simulink model "soc_rfsoc_fpga"  (R2025b)
settings: Solver=FixedStepDiscrete  StartTime=0.0  StopTime=15e-4  RelTol=1e-3
undefined symbols (not defined in the file): downSamplingFactor, SampleTime
libraries: simulink x4, hdlsllib x3, hwlogicconnlib x2, dspsrcs4 x2, socmemlib x1
settings Model: DataTypeOverride=Off  Creator=The MathWorks, Inc.  LastModifiedBy=The MathWorks, Inc.
settings SolverCC: AlgebraicLoopSolver=TrustRegion  PositivePriorityOrder=on  MaxZcPerStep=1.0
settings DataIOCC: SaveOutput=off  SaveTime=off  ReturnWorkspaceOutputs=off
settings OptimizationCC: BlockReduction=off  ConditionallyExecuteInputs=off  DefaultParameterBehavior=Inlined  PassReuseOutputArgsAs=Individual arguments  MaxStackSize=64  EfficientTunableParamExpr=on
settings DebuggingCC: AlgebraicLoopMsg=error  SingleTaskRateTransMsg=error  IntegerOverflowMsg=none  ParameterPrecisionLossMsg=none  ParameterTunabilityLossMsg=error  UnconnectedInputMsg=warning  UnconnectedOutputMsg=warning  UnconnectedLineMsg=warning  PregeneratedLibrarySubsystemCodeDiagnostic=none  SFUnexpectedBacktrackingDiag=warning  SFNoUnconditionalDefaultTransitionDiag=warning  ArithmeticOperatorsInVariantConditions=warning
settings HardwareCC: ProdBitPerPointer=32.0  ProdBitPerSizeT=32.0  ProdBitPerPtrDiffT=32.0  ProdLargestAtomicFloat=None  ProdIntDivRoundTo=Undefined  ProdEndianess=Unspecified  ProdWordSize=32.0  ProdHWDeviceType=ASIC/FPGA->ASIC/FPGA  TargetBitPerLong=64.0  TargetBitPerPointer=64.0  TargetBitPerSizeT=64.0  TargetBitPerPtrDiffT=64.0  TargetLongLongMode=on  TargetIntDivRoundTo=Zero  TargetEndianess=LittleEndian  TargetWordSize=64.0  TargetHWDeviceType=Custom Processor->MATLAB Host Computer  ProdEqTarget=off  HardwareBoardFeatureSet=SoCBlockset
settings ModelReferenceCC: EnableRefExpFcnMdlSchedulingChecks=on  ModelReferenceNumInstancesAllowed=Single
settings SFSimCC: SimUseLocalCustomCode=off
settings RTWCC: SystemTargetFile=ert.tlc  HardwareBoard=Xilinx Zynq UltraScale+ RFSoC ZCU111 Evaluation Kit  TLCOptions="-aInlineSetEventsForThisBaseRateFcn=TLC_FALSE -aSuppressMultiTaskScheduler=TLC_FALSE  -aRateBasedStepFcn=0"  TemplateMakefile=ert_default_tmf  GenerateReport=on  RTWUseLocalCustomCode=off  Toolchain=Linaro AArch64 Linux v6.3.1  IncludeHyperlinkInReport=on  LaunchReport=on  GenerateTraceInfo=on  GenerateTraceReport=on  GenerateTraceReportSl=on  GenerateTraceReportSf=on  GenerateTraceReportEml=on  GPUComputeCapability=3.5  DLArmComputeVersion=19.05  Description=Embedded Coder
settings CodeAppCC: ForceParamTrailComments=on  IgnoreCustomStorageClasses=off  OperatorAnnotations=on  SimulinkDataObjDesc=on  SFDataObjDesc=on  InsertBlockDesc=on
settings ERTTargetCC: InlinedParameterPlacement=Hierarchical  DynamicArrayContainerType=coder::array  SubcomponentCodeInterfacePackaging=Nonreusable function

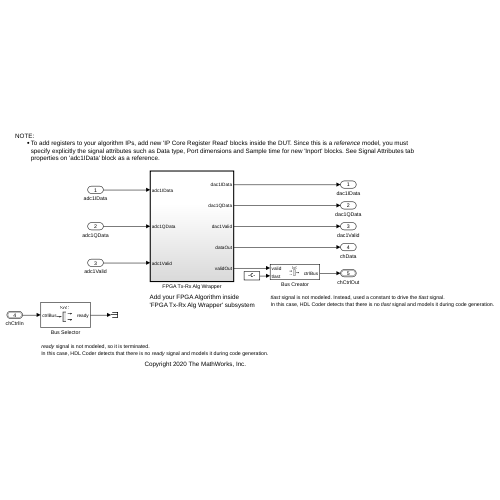
[thumbnail: Simulink's stored preview of the top-level diagram]
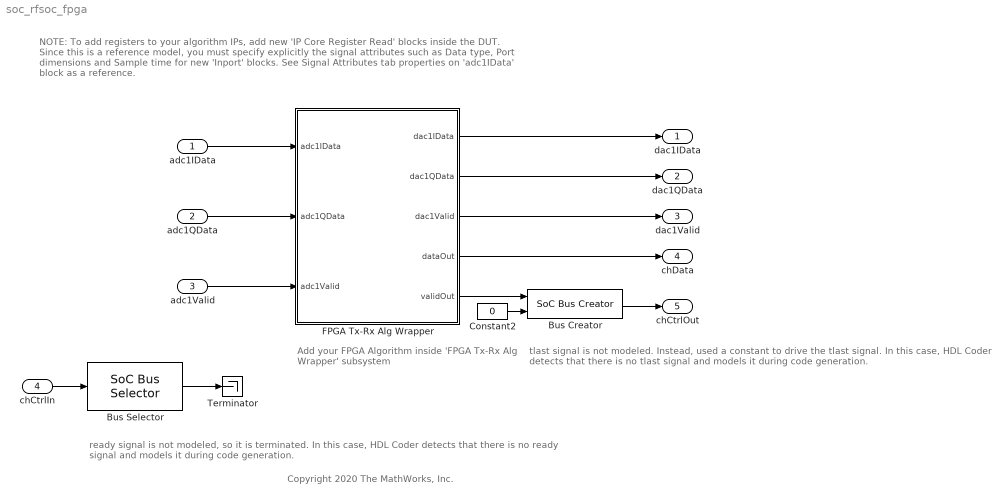
== system soc_rfsoc_fpga ==
  note: Add your FPGA Algorithm inside
      | 'FPGA Tx-Rx Alg Wrapper' subsystem
  note: NOTE:
      | To add registers to your algorithm IPs, add new 'IP Core Register Read' blocks inside the DUT. Since this is a reference model, you must specify explicitly the signal attributes such as Data type, Port dimensions and Sample time for new 'Inport' blocks. See Signal Attributes tab properties on 'adc1IData' block as a reference.
  note: Copyright 2020 The MathWorks, Inc.
  note: ready signal is not modeled, so it is terminated.
      | In this case, HDL Coder detects that there is no ready signal and models it during code generation.
  note: tlast signal is not modeled. Instead, used a constant to drive the tlast signal.
      | In this case, HDL Coder detects that there is no tlast signal and models it during code generation.
  adc1IData : Inport  OutDataTypeStr=int16  PortDimensions=2  SampleTime=SampleTime
  adc1QData : Inport  Port=2  OutDataTypeStr=int16  PortDimensions=2
  adc1Valid : Inport  Port=3  OutDataTypeStr=boolean
  chCtrlIn : Inport  Port=4  OutDataTypeStr=Bus: StreamS2MBusObj  BusOutputAsStruct=on
  Bus Creator : hwlogicconnlib/SoC Bus Creator  Protocol=Data stream  ctrltype=Valid
  Bus Selector : hwlogicconnlib/SoC Bus Selector  Protocol=Data stream  ctrltype=Ready
  Constant2 : Constant  Value=0  OutDataTypeStr=boolean  SampleTime=-1
  FPGA Tx-Rx Alg Wrapper : Subsystem  TreatAsAtomicUnit=on
  Terminator : Terminator
  dac1IData : Outport  VectorParamsAs1DForOutWhenUnconnected=off
  dac1QData : Outport  Port=2  VectorParamsAs1DForOutWhenUnconnected=off
  dac1Valid : Outport  Port=3  VectorParamsAs1DForOutWhenUnconnected=off
  chData : Outport  Port=4  VectorParamsAs1DForOutWhenUnconnected=off
  chCtrlOut : Outport  Port=5  OutDataTypeStr=Bus: StreamM2SBusObj  VectorParamsAs1DForOutWhenUnconnected=off  BusOutputAsStruct=on
  wires:
  adc1QData/1 -> FPGA Tx-Rx Alg Wrapper/2(adc1QData)
  FPGA Tx-Rx Alg Wrapper/5(validOut) -> Bus Creator/1
  adc1IData/1 -> FPGA Tx-Rx Alg Wrapper/1(adc1IData)
  Bus Creator/1 -> chCtrlOut/1
  Constant2/1 -> Bus Creator/2
  chCtrlIn/1 -> Bus Selector/1
  Bus Selector/1 -> Terminator/1
  FPGA Tx-Rx Alg Wrapper/1(dac1IData) -> dac1IData/1
  FPGA Tx-Rx Alg Wrapper/2(dac1QData) -> dac1QData/1
  FPGA Tx-Rx Alg Wrapper/3(dac1Valid) -> dac1Valid/1
  FPGA Tx-Rx Alg Wrapper/4(dataOut) -> chData/1
  adc1Valid/1 -> FPGA Tx-Rx Alg Wrapper/3(adc1Valid)

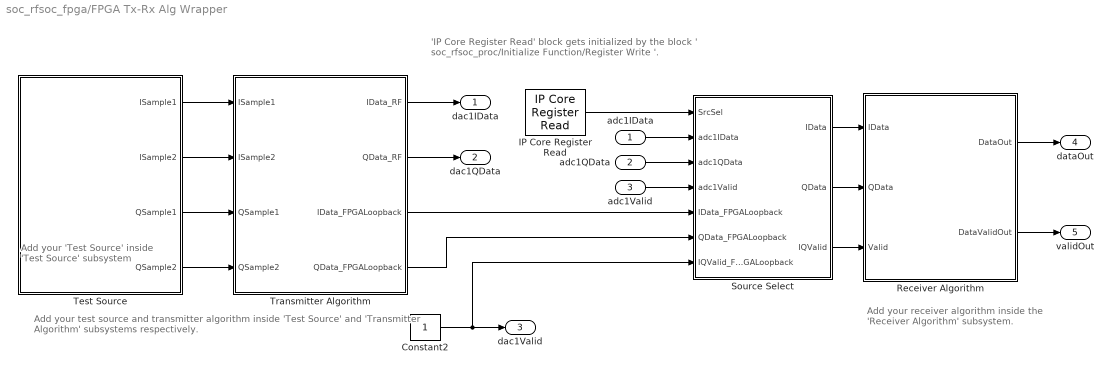
== system soc_rfsoc_fpga/FPGA Tx-Rx Alg Wrapper ==
  note: Add your receiver algorithm inside
      | the 'Receiver Algorithm' subsystem.
  note: Add your 'Test Source' inside
      | 'Test Source' subsystem
  note: Add your test source and transmitter algorithm inside
      | 'Test Source' and 'Transmitter Algorithm' subsystems respectively.
  note: 'IP Core Register Read' block gets initialized by the block
      | ' soc_rfsoc_proc/Initialize Function/Register Write '.
  adc1IData : Inport
  adc1QData : Inport  Port=2
  adc1Valid : Inport  Port=3
  Constant2 : Constant  OutDataTypeStr=boolean  SampleTime=-1
  IP Core Register Read : socmemlib/IP Core Register Read  RegisterName=SrcSelReg  OutDataTypeStr=boolean  OutputVectorSize=1  SampleTime=SampleTime
  Receiver Algorithm : Subsystem
  Source Select : Subsystem
  Test Source : Subsystem  TreatAsAtomicUnit=on
  Transmitter Algorithm : Subsystem  TreatAsAtomicUnit=on
  dac1IData : Outport  VectorParamsAs1DForOutWhenUnconnected=off
  dac1QData : Outport  Port=2  VectorParamsAs1DForOutWhenUnconnected=off
  dac1Valid : Outport  Port=3  VectorParamsAs1DForOutWhenUnconnected=off
  dataOut : Outport  Port=4  VectorParamsAs1DForOutWhenUnconnected=off
  validOut : Outport  Port=5  VectorParamsAs1DForOutWhenUnconnected=off
  wires:
  Receiver Algorithm/1(DataOut) -> dataOut/1
  Receiver Algorithm/2(DataValidOut) -> validOut/1
  Constant2/1 -> Source Select/7(IQValid_FPGALoopback), dac1Valid/1
  Transmitter Algorithm/1(IData_RF) -> dac1IData/1
  Transmitter Algorithm/2(QData_RF) -> dac1QData/1
  Test Source/1(ISample1) -> Transmitter Algorithm/1(ISample1)
  Test Source/2(ISample2) -> Transmitter Algorithm/2(ISample2)
  Test Source/3(QSample1) -> Transmitter Algorithm/3(QSample1)
  Test Source/4(QSample2) -> Transmitter Algorithm/4(QSample2)
  IP Core Register Read/1 -> Source Select/1(SrcSel)
  adc1IData/1 -> Source Select/2(adc1IData)
  Transmitter Algorithm/3(IData_FPGALoopback) -> Source Select/5(IData_FPGALoopback)
  adc1QData/1 -> Source Select/3(adc1QData)
  Transmitter Algorithm/4(QData_FPGALoopback) -> Source Select/6(QData_FPGALoopback)
  adc1Valid/1 -> Source Select/4(adc1Valid)
  Source Select/1(IData) -> Receiver Algorithm/1(IData)
  Source Select/2(QData) -> Receiver Algorithm/2(QData)
  Source Select/3(IQValid) -> Receiver Algorithm/3(Valid)

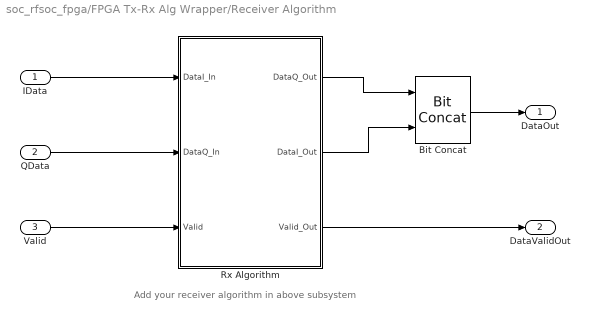
== system soc_rfsoc_fpga/FPGA Tx-Rx Alg Wrapper/Receiver Algorithm ==
  note: Add your receiver algorithm in above subsystem
  IData : Inport
  QData : Inport  Port=2
  Valid : Inport  Port=3
  Bit Concat : hdlsllib/Logic and Bit Operations/Bit Concat  numInputs=2
  Rx Algorithm : Subsystem
  DataOut : Outport  VectorParamsAs1DForOutWhenUnconnected=off
  DataValidOut : Outport  Port=2  VectorParamsAs1DForOutWhenUnconnected=off
  wires:
  Rx Algorithm/3(Valid_Out) -> DataValidOut/1
  QData/1 -> Rx Algorithm/2(DataQ_In)
  Bit Concat/1 -> DataOut/1
  Valid/1 -> Rx Algorithm/3(Valid)
  IData/1 -> Rx Algorithm/1(DataI_In)
  Rx Algorithm/1(DataQ_Out) -> Bit Concat/1
  Rx Algorithm/2(DataI_Out) -> Bit Concat/2

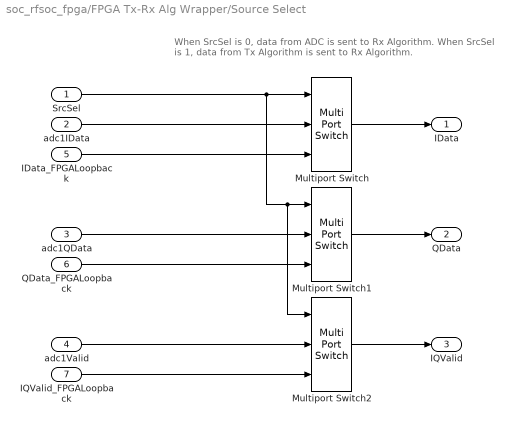
== system soc_rfsoc_fpga/FPGA Tx-Rx Alg Wrapper/Source Select ==
  note: When SrcSel is 0, data from ADC is sent to Rx Algorithm.
      | When SrcSel is 1, data from Tx Algorithm is sent to Rx Algorithm.
  SrcSel : Inport
  adc1IData : Inport  Port=2
  adc1QData : Inport  Port=3
  adc1Valid : Inport  Port=4
  IData_FPGALoopback : Inport  Port=5
  QData_FPGALoopback : Inport  Port=6
  IQValid_FPGALoopback : Inport  Port=7
  Multiport Switch : MultiPortSwitch  DataPortOrder=Zero-based contiguous  Inputs=2  zeroidx=on  SaturateOnIntegerOverflow=off  InputSameDT=off
  Multiport Switch1 : MultiPortSwitch  DataPortOrder=Zero-based contiguous  Inputs=2  zeroidx=on  SaturateOnIntegerOverflow=off  InputSameDT=off
  Multiport Switch2 : MultiPortSwitch  DataPortOrder=Zero-based contiguous  Inputs=2  zeroidx=on  SaturateOnIntegerOverflow=off  InputSameDT=off
  IData : Outport
  QData : Outport  Port=2
  IQValid : Outport  Port=3
  wires:
  IQValid_FPGALoopback/1 -> Multiport Switch2/3
  SrcSel/1 -> Multiport Switch2/1, Multiport Switch1/1, Multiport Switch/1
  adc1Valid/1 -> Multiport Switch2/2
  Multiport Switch1/1 -> QData/1
  Multiport Switch/1 -> IData/1
  QData_FPGALoopback/1 -> Multiport Switch1/3
  adc1QData/1 -> Multiport Switch1/2
  Multiport Switch2/1 -> IQValid/1
  IData_FPGALoopback/1 -> Multiport Switch/3
  adc1IData/1 -> Multiport Switch/2

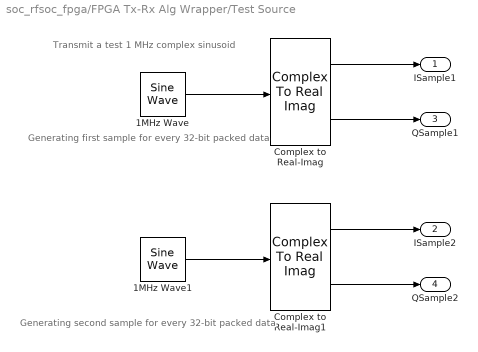
== system soc_rfsoc_fpga/FPGA Tx-Rx Alg Wrapper/Test Source ==
  note: Transmit a test 1 MHz complex sinusoid
  note: Generating first sample for every 32-bit packed data
  note: Generating second sample for every 32-bit packed data
  1MHz Wave : dspsrcs4/Sine Wave  Amplitude=2^14  Frequency=1e6  Phase=0  SampleMode=Discrete  OutComplex=Complex  CompMethod=Table lookup  TableSize=Speed  SampleTime=SampleTime  SamplesPerFrame=1  ResetState=Restart at time zero  OutputFrames=off  dataType=Fixed-point  wordLen=16  udDataType=sfix(16)  fracBitsMode=User-defined  numFracBits=0  OutDataTypeStr=fixdt(1,16,0)  LastOutDataTypeStr=fixdt(1,16,0)
  1MHz Wave1 : dspsrcs4/Sine Wave  Amplitude=2^14  Frequency=1e6  Phase=pi/128  SampleMode=Discrete  OutComplex=Complex  CompMethod=Table lookup  TableSize=Speed  SampleTime=SampleTime  SamplesPerFrame=1  ResetState=Restart at time zero  OutputFrames=off  dataType=Fixed-point  wordLen=16  udDataType=sfix(16)  fracBitsMode=User-defined  numFracBits=0  OutDataTypeStr=fixdt(1,16,0)  LastOutDataTypeStr=fixdt(1,16,0)
  Complex to Real-Imag : ComplexToRealImag
  Complex to Real-Imag1 : ComplexToRealImag
  ISample1 : Outport
  ISample2 : Outport  Port=2
  QSample1 : Outport  Port=3
  QSample2 : Outport  Port=4
  wires:
  1MHz Wave/1 -> Complex to Real-Imag/1
  1MHz Wave1/1 -> Complex to Real-Imag1/1
  Complex to Real-Imag/1 -> ISample1/1
  Complex to Real-Imag1/1 -> ISample2/1
  Complex to Real-Imag/2 -> QSample1/1
  Complex to Real-Imag1/2 -> QSample2/1

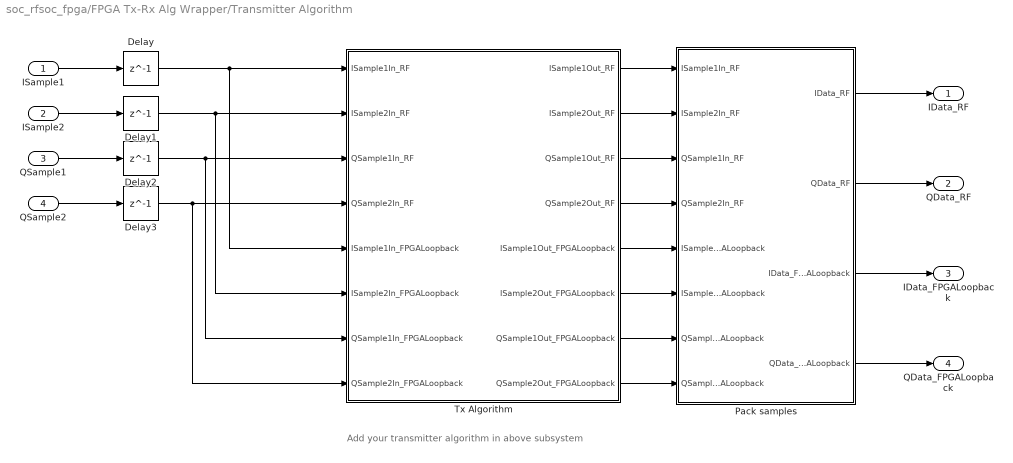
== system soc_rfsoc_fpga/FPGA Tx-Rx Alg Wrapper/Transmitter Algorithm ==
  note: Add your transmitter algorithm in above subsystem
  ISample1 : Inport
  ISample2 : Inport  Port=2
  QSample1 : Inport  Port=3
  QSample2 : Inport  Port=4
  Delay{,1..3} (4 alike) : Delay  DelayLength=1  InitialCondition=0
  Pack samples : Subsystem
  Tx Algorithm : Subsystem
  IData_RF : Outport  VectorParamsAs1DForOutWhenUnconnected=off
  QData_RF : Outport  Port=2  VectorParamsAs1DForOutWhenUnconnected=off
  IData_FPGALoopback : Outport  Port=3  VectorParamsAs1DForOutWhenUnconnected=off
  QData_FPGALoopback : Outport  Port=4  VectorParamsAs1DForOutWhenUnconnected=off
  wires:
  ISample1/1 -> Delay/1
  ISample2/1 -> Delay1/1
  Delay/1 -> Tx Algorithm/5(ISample1In_FPGALoopback), Tx Algorithm/1(ISample1In_RF)
  Delay1/1 -> Tx Algorithm/6(ISample2In_FPGALoopback), Tx Algorithm/2(ISample2In_RF)
  QSample1/1 -> Delay2/1
  QSample2/1 -> Delay3/1
  Delay2/1 -> Tx Algorithm/7(QSample1In_FPGALoopback), Tx Algorithm/3(QSample1In_RF)
  Delay3/1 -> Tx Algorithm/8(QSample2In_FPGALoopback), Tx Algorithm/4(QSample2In_RF)
  Tx Algorithm/1(ISample1Out_RF) -> Pack samples/1(ISample1In_RF)
  Tx Algorithm/2(ISample2Out_RF) -> Pack samples/2(ISample2In_RF)
  Tx Algorithm/3(QSample1Out_RF) -> Pack samples/3(QSample1In_RF)
  Tx Algorithm/4(QSample2Out_RF) -> Pack samples/4(QSample2In_RF)
  Tx Algorithm/5(ISample1Out_FPGALoopback) -> Pack samples/5(ISample1In_FPGALoopback)
  Tx Algorithm/6(ISample2Out_FPGALoopback) -> Pack samples/6(ISample2In_FPGALoopback)
  Tx Algorithm/7(QSample1Out_FPGALoopback) -> Pack samples/7(QSample1In_FPGALoopback)
  Tx Algorithm/8(QSample2Out_FPGALoopback) -> Pack samples/8(QSample2In_FPGALoopback)
  Pack samples/1(IData_RF) -> IData_RF/1
  Pack samples/3(IData_FPGALoopback) -> IData_FPGALoopback/1
  Pack samples/4(QData_FPGALoopback) -> QData_FPGALoopback/1
  Pack samples/2(QData_RF) -> QData_RF/1

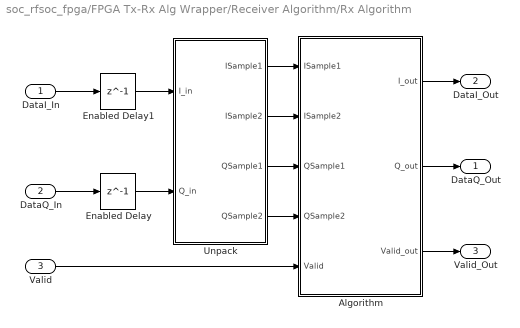
== system soc_rfsoc_fpga/FPGA Tx-Rx Alg Wrapper/Receiver Algorithm/Rx Algorithm ==
  DataI_In : Inport
  DataQ_In : Inport  Port=2
  Valid : Inport  Port=3
  Algorithm : Subsystem
  Enabled Delay : Delay  DelayLength=1
  Enabled Delay1 : Delay  DelayLength=1
  Unpack : Subsystem
  DataQ_Out : Outport  VectorParamsAs1DForOutWhenUnconnected=off
  DataI_Out : Outport  Port=2  VectorParamsAs1DForOutWhenUnconnected=off
  Valid_Out : Outport  Port=3  VectorParamsAs1DForOutWhenUnconnected=off
  wires:
  Unpack/1(ISample1) -> Algorithm/1(ISample1)
  Algorithm/3(Valid_out) -> Valid_Out/1
  DataI_In/1 -> Enabled Delay1/1
  Algorithm/1(I_out) -> DataI_Out/1
  Unpack/4(QSample2) -> Algorithm/4(QSample2)
  Algorithm/2(Q_out) -> DataQ_Out/1
  Unpack/2(ISample2) -> Algorithm/2(ISample2)
  Enabled Delay/1 -> Unpack/2(Q_in)
  Unpack/3(QSample1) -> Algorithm/3(QSample1)
  Enabled Delay1/1 -> Unpack/1(I_in)
  Valid/1 -> Algorithm/5(Valid)
  DataQ_In/1 -> Enabled Delay/1

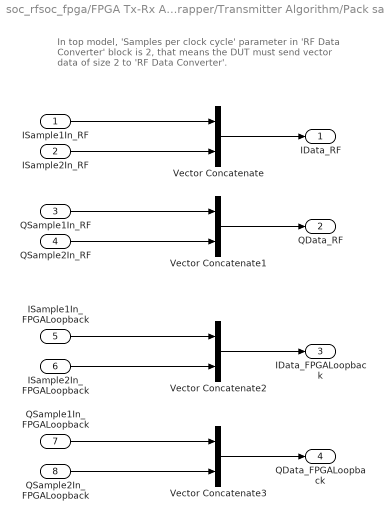
== system soc_rfsoc_fpga/FPGA Tx-Rx Alg Wrapper/Transmitter Algorithm/Pack samples ==
  note: In top model, 'Samples per clock cycle' parameter in 'RF
      | Data Converter' block is 2, that means the DUT must send
      | vector data of size 2 to 'RF Data Converter'.
  ISample1In_RF : Inport
  ISample2In_RF : Inport  Port=2
  QSample1In_RF : Inport  Port=3
  QSample2In_RF : Inport  Port=4
  ISample1In_FPGALoopback : Inport  Port=5
  ISample2In_FPGALoopback : Inport  Port=6
  QSample1In_FPGALoopback : Inport  Port=7
  QSample2In_FPGALoopback : Inport  Port=8
  Vector Concatenate{,1..3} (4 alike) : Concatenate
  IData_RF : Outport  VectorParamsAs1DForOutWhenUnconnected=off
  QData_RF : Outport  Port=2  VectorParamsAs1DForOutWhenUnconnected=off
  IData_FPGALoopback : Outport  Port=3  VectorParamsAs1DForOutWhenUnconnected=off
  QData_FPGALoopback : Outport  Port=4  VectorParamsAs1DForOutWhenUnconnected=off
  wires:
  Vector Concatenate1/1 -> QData_RF/1
  Vector Concatenate2/1 -> IData_FPGALoopback/1
  Vector Concatenate3/1 -> QData_FPGALoopback/1
  ISample2In_RF/1 -> Vector Concatenate/2
  ISample1In_RF/1 -> Vector Concatenate/1
  QSample2In_RF/1 -> Vector Concatenate1/2
  QSample1In_RF/1 -> Vector Concatenate1/1
  ISample2In_FPGALoopback/1 -> Vector Concatenate2/2
  ISample1In_FPGALoopback/1 -> Vector Concatenate2/1
  QSample2In_FPGALoopback/1 -> Vector Concatenate3/2
  QSample1In_FPGALoopback/1 -> Vector Concatenate3/1
  Vector Concatenate/1 -> IData_RF/1

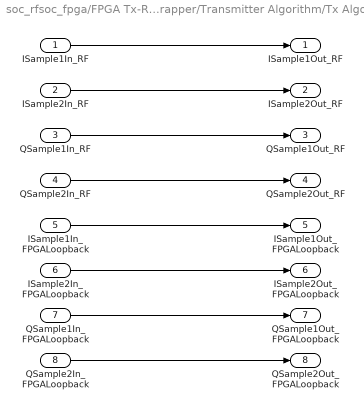
== system soc_rfsoc_fpga/FPGA Tx-Rx Alg Wrapper/Transmitter Algorithm/Tx Algorithm ==
  ISample1In_RF : Inport
  ISample2In_RF : Inport  Port=2
  QSample1In_RF : Inport  Port=3
  QSample2In_RF : Inport  Port=4
  ISample1In_FPGALoopback : Inport  Port=5
  ISample2In_FPGALoopback : Inport  Port=6
  QSample1In_FPGALoopback : Inport  Port=7
  QSample2In_FPGALoopback : Inport  Port=8
  ISample1Out_RF : Outport  VectorParamsAs1DForOutWhenUnconnected=off
  ISample2Out_RF : Outport  Port=2  VectorParamsAs1DForOutWhenUnconnected=off
  QSample1Out_RF : Outport  Port=3  VectorParamsAs1DForOutWhenUnconnected=off
  QSample2Out_RF : Outport  Port=4  VectorParamsAs1DForOutWhenUnconnected=off
  ISample1Out_FPGALoopback : Outport  Port=5  VectorParamsAs1DForOutWhenUnconnected=off
  ISample2Out_FPGALoopback : Outport  Port=6  VectorParamsAs1DForOutWhenUnconnected=off
  QSample1Out_FPGALoopback : Outport  Port=7  VectorParamsAs1DForOutWhenUnconnected=off
  QSample2Out_FPGALoopback : Outport  Port=8  VectorParamsAs1DForOutWhenUnconnected=off
  wires:
  ISample1In_RF/1 -> ISample1Out_RF/1
  ISample2In_RF/1 -> ISample2Out_RF/1
  ISample1In_FPGALoopback/1 -> ISample1Out_FPGALoopback/1
  ISample2In_FPGALoopback/1 -> ISample2Out_FPGALoopback/1
  QSample2In_RF/1 -> QSample2Out_RF/1
  QSample1In_RF/1 -> QSample1Out_RF/1
  QSample2In_FPGALoopback/1 -> QSample2Out_FPGALoopback/1
  QSample1In_FPGALoopback/1 -> QSample1Out_FPGALoopback/1

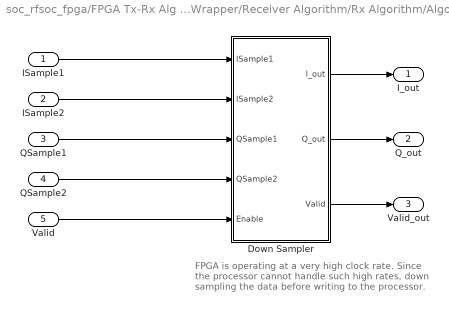
== system soc_rfsoc_fpga/FPGA Tx-Rx Alg Wrapper/Receiver Algorithm/Rx Algorithm/Algorithm ==
  note: FPGA is operating at a very high clock rate. Since the processor cannot handle such high rates, down sampling
      | the data before writing to the processor.
  ISample1 : Inport
  ISample2 : Inport  Port=2
  QSample1 : Inport  Port=3
  QSample2 : Inport  Port=4
  Valid : Inport  Port=5
  Down Sampler : Subsystem
  I_out : Outport  VectorParamsAs1DForOutWhenUnconnected=off
  Q_out : Outport  Port=2  VectorParamsAs1DForOutWhenUnconnected=off
  Valid_out : Outport  Port=3  VectorParamsAs1DForOutWhenUnconnected=off
  wires:
  Valid/1 -> Down Sampler/5(Enable)
  Down Sampler/3(Valid) -> Valid_out/1
  QSample1/1 -> Down Sampler/3(QSample1)
  ISample1/1 -> Down Sampler/1(ISample1)
  Down Sampler/2(Q_out) -> Q_out/1
  Down Sampler/1(I_out) -> I_out/1
  ISample2/1 -> Down Sampler/2(ISample2)
  QSample2/1 -> Down Sampler/4(QSample2)

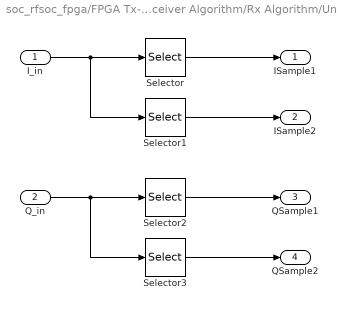
== system soc_rfsoc_fpga/FPGA Tx-Rx Alg Wrapper/Receiver Algorithm/Rx Algorithm/Unpack ==
  I_in : Inport
  Q_in : Inport  Port=2
  Selector : Selector  InputPortWidth=2  IndexOptions=Index vector (dialog)  Indices=1  OutputSizes=1
  Selector1 : Selector  InputPortWidth=2  IndexOptions=Index vector (dialog)  Indices=2  OutputSizes=1
  Selector2 : Selector  InputPortWidth=2  IndexOptions=Index vector (dialog)  Indices=1  OutputSizes=1
  Selector3 : Selector  InputPortWidth=2  IndexOptions=Index vector (dialog)  Indices=2  OutputSizes=1
  ISample1 : Outport
  ISample2 : Outport  Port=2
  QSample1 : Outport  Port=3
  QSample2 : Outport  Port=4
  wires:
  Selector/1 -> ISample1/1
  Selector2/1 -> QSample1/1
  Selector1/1 -> ISample2/1
  Q_in/1 -> Selector3/1, Selector2/1
  I_in/1 -> Selector1/1, Selector/1
  Selector3/1 -> QSample2/1

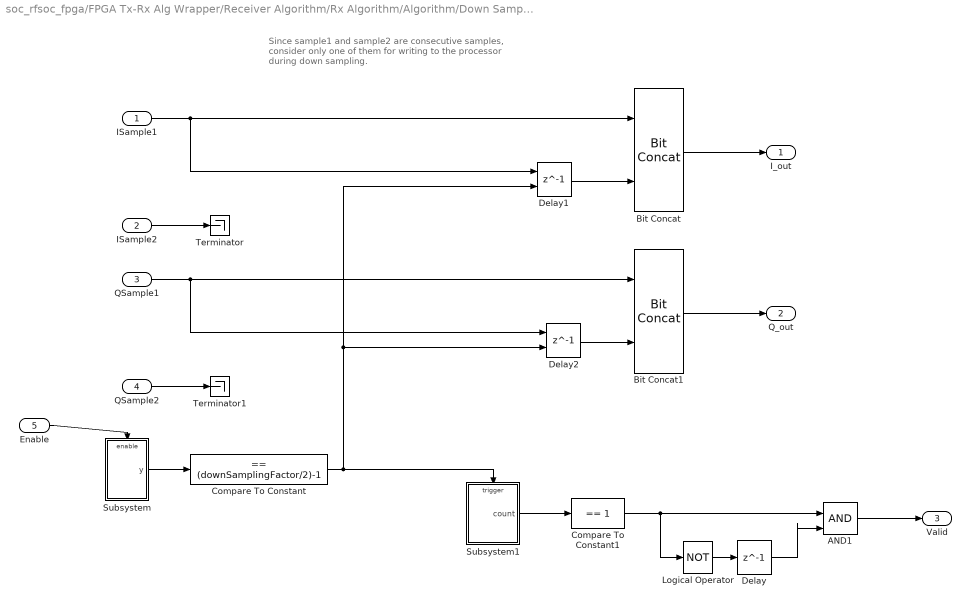
== system soc_rfsoc_fpga/FPGA Tx-Rx Alg Wrapper/Receiver Algorithm/Rx Algorithm/Algorithm/Down Sampler ==
  note: Since sample1 and sample2 are consecutive samples,
      | consider only one of them for writing to the processor
      | during down sampling.
  ISample1 : Inport
  ISample2 : Inport  Port=2
  QSample1 : Inport  Port=3
  QSample2 : Inport  Port=4
  Enable : Inport  Port=5
  AND1 : Logic  IconShape=distinctive  AllPortsSameDT=off  OutDataTypeStr=boolean
  Bit Concat : hdlsllib/Logic and Bit Operations/Bit Concat  numInputs=2
  Bit Concat1 : hdlsllib/Logic and Bit Operations/Bit Concat  numInputs=2
  Compare To Constant : simulink/Logic and Bit Operations/Compare To Constant  relop===  const=(downSamplingFactor/2)-1  OutDataTypeStr=boolean
  Compare To Constant1 : simulink/Logic and Bit Operations/Compare To Constant  relop===  const=1  OutDataTypeStr=boolean
  Delay : Delay  DelayLength=1
  Delay1 : Delay  DelayLength=1  ShowEnablePort=on
      settings: InputPortMap=u0,e6
  Delay2 : Delay  DelayLength=1  ShowEnablePort=on
      settings: InputPortMap=u0,e6
  Logical Operator : Logic  Operator=NOT  IconShape=distinctive  AllPortsSameDT=off  OutDataTypeStr=boolean
  Subsystem : Subsystem
  Subsystem1 : Subsystem
  Terminator : Terminator
  Terminator1 : Terminator
  I_out : Outport  VectorParamsAs1DForOutWhenUnconnected=off
  Q_out : Outport  Port=2  VectorParamsAs1DForOutWhenUnconnected=off
  Valid : Outport  Port=3
  wires:
  Enable/1 -> Subsystem/Enable
  Subsystem/1(y) -> Compare To Constant/1
  Compare To Constant1/1 -> AND1/1, Logical Operator/1
  Compare To Constant/1 -> Subsystem1/Trigger, Delay1/2, Delay2/2
  Logical Operator/1 -> Delay/1
  AND1/1 -> Valid/1
  ISample1/1 -> Bit Concat/1, Delay1/1
  Delay/1 -> AND1/2
  Subsystem1/1(count) -> Compare To Constant1/1
  QSample1/1 -> Bit Concat1/1, Delay2/1
  Bit Concat/1 -> I_out/1
  Bit Concat1/1 -> Q_out/1
  Delay1/1 -> Bit Concat/2
  Delay2/1 -> Bit Concat1/2
  ISample2/1 -> Terminator/1
  QSample2/1 -> Terminator1/1

== system soc_rfsoc_fpga/FPGA Tx-Rx Alg Wrapper/Receiver Algorithm/Rx Algorithm/Algorithm/Down Sampler/Subsystem ==
  Enable : EnablePort
  Counter Limited : simulink/Sources/Counter Limited  uplimit=(downSamplingFactor/2)-1  tsamp=-1
  y : Outport  InitialOutput=0
  wires:
  Counter Limited/1 -> y/1

== system soc_rfsoc_fpga/FPGA Tx-Rx Alg Wrapper/Receiver Algorithm/Rx Algorithm/Algorithm/Down Sampler/Subsystem1 ==
  Trigger : TriggerPort  VariantControl=Variant  PortDimensions=1
  Counter Limited : simulink/Sources/Counter Limited  uplimit=1  tsamp=-1
  count : Outport  InitialOutput=0
  wires:
  Counter Limited/1 -> count/1
